simulink subsystem "rho_ideal"  (R2020a)
settings: Solver=VariableStepAuto  StartTime=0.0  StopTime=10.0  RelTol=1e-3
settings Model: Creator=Philip  LastModifiedBy=Philip

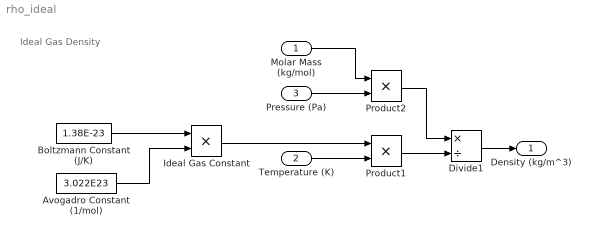
== system rho_ideal ==
  note: Ideal Gas Density
  Molar Mass (kg/mol) : Inport
  Temperature (K) : Inport  Port=2
  Pressure (Pa) : Inport  Port=3
  Avogadro Constant (1/mol) : Constant  Value=3.022E23
  Boltzmann Constant (J/K) : Constant  Value=1.38E-23
  Divide1 : Product  Inputs=*/
  Ideal Gas Constant : Product
  Product1 : Product
  Product2 : Product
  Density (kg/m^3) : Outport
  wires:
  Product2/1 -> Divide1/1
  Product1/1 -> Divide1/2
  Divide1/1 -> Density (kg/m^3)/1
  Temperature (K)/1 -> Product1/2
  Ideal Gas Constant/1 -> Product1/1
  Pressure (Pa)/1 -> Product2/2
  Molar Mass (kg/mol)/1 -> Product2/1
  Boltzmann Constant (J/K)/1 -> Ideal Gas Constant/1
  Avogadro Constant (1/mol)/1 -> Ideal Gas Constant/2
